simulink model "PasiveBalancer20S"  (R2021a)
settings: Solver=VariableStepAuto  StartTime=0.0  StopTime=30000  RelTol=1e-3
undefined symbols (not defined in the file): Ion, Lithium
libraries: spsIdealSwitchLib x22, spsSeriesRLCBranchLib x21, spsBatteryLib x20, spsDCVoltageSourceLib x1, spspowerguiLib x1
settings Model: SimulationMode=rapid-accelerator  Creator=jafar  LastModifiedBy=jafar
settings SolverCC: ZeroCrossAlgorithm=Adaptive
settings DebuggingCC: IgnoredZcDiagnostic=none

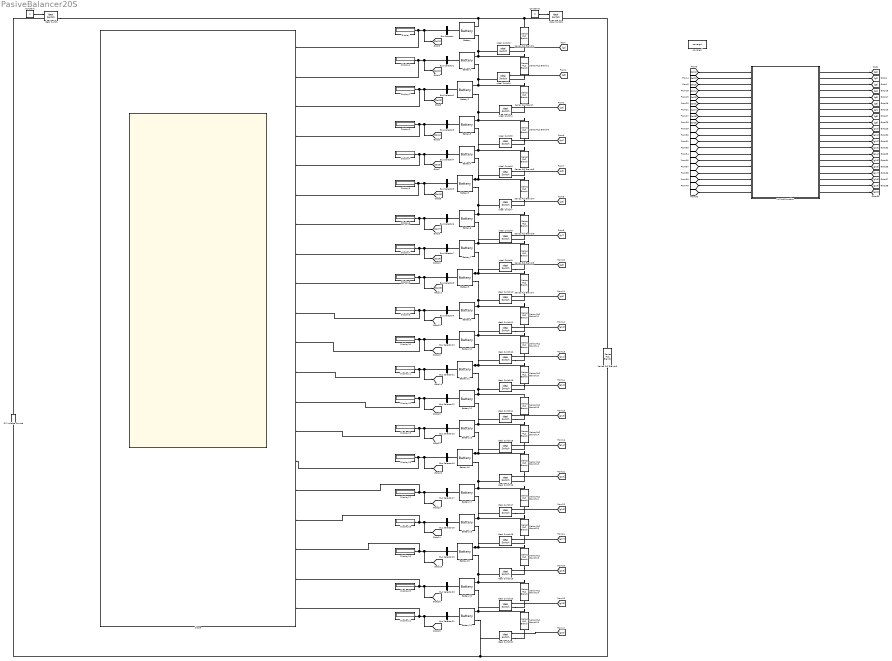
== system PasiveBalancer20S ==
  Battery : spsBatteryLib/Battery  BatType=Lithium-Ion  ShowTempParam=off  ThermalPreset=no  ShowAgeParam=off  NomV=3.7  NomQ=30  SOC=20  Batt_Tr=30  PresetModel=on  MaxQ=30  MinV=2.775  FullV=4.3068  Dis_rate=13.0435  R=0.0012333  Normal_OP=27.1304  expZone="[3.9974      1.4739]"  current=[6.5 13 32.5]  Units=Time  Tci=20  NomT=20  T2=-30  MaxQ2=4.8  FullV2=7.1  Normal_OP2=5.655  expZone2="[6.58           1]"  Rca=0.6  ti=2000  Dp=0  Neq0=0  Tsim=1e6  Ta1=25  Qeol=5.4*0.9  Reol=0.013333*1.2  Char_age=[2.3478, 3]  Dis_age=[2.3478, 10]  N1=1500  N2=10500  N3=1000  N4=1400  Ta2=45  N5=950
  Battery1 : spsBatteryLib/Battery  BatType=Lithium-Ion  ShowTempParam=off  ThermalPreset=no  ShowAgeParam=off  NomV=3.7  NomQ=30  SOC=23  Batt_Tr=30  PresetModel=on  MaxQ=30  MinV=2.775  FullV=4.3068  Dis_rate=13.0435  R=0.0012333  Normal_OP=27.1304  expZone="[3.9974      1.4739]"  current=[6.5 13 32.5]  Units=Time  Tci=20  NomT=20  T2=-30  MaxQ2=4.8  FullV2=7.1  Normal_OP2=5.655  expZone2="[6.58           1]"  Rca=0.6  ti=2000  Dp=0  Neq0=0  Tsim=1e6  Ta1=25  Qeol=5.4*0.9  Reol=0.013333*1.2  Char_age=[2.3478, 3]  Dis_age=[2.3478, 10]  N1=1500  N2=10500  N3=1000  N4=1400  Ta2=45  N5=950
  Battery10 : spsBatteryLib/Battery  BatType=Lithium-Ion  ShowTempParam=off  ThermalPreset=no  ShowAgeParam=off  NomV=3.7  NomQ=30  SOC=50  Batt_Tr=30  PresetModel=on  MaxQ=30  MinV=2.775  FullV=4.3068  Dis_rate=13.0435  R=0.0012333  Normal_OP=27.1304  expZone="[3.9974      1.4739]"  current=[6.5 13 32.5]  Units=Time  Tci=20  NomT=20  T2=-30  MaxQ2=4.8  FullV2=7.1  Normal_OP2=5.655  expZone2="[6.58           1]"  Rca=0.6  ti=2000  Dp=0  Neq0=0  Tsim=1e6  Ta1=25  Qeol=5.4*0.9  Reol=0.013333*1.2  Char_age=[2.3478, 3]  Dis_age=[2.3478, 10]  N1=1500  N2=10500  N3=1000  N4=1400  Ta2=45  N5=950
  Battery11 : spsBatteryLib/Battery  BatType=Lithium-Ion  ShowTempParam=off  ThermalPreset=no  ShowAgeParam=off  NomV=3.7  NomQ=30  SOC=53  Batt_Tr=30  PresetModel=on  MaxQ=30  MinV=2.775  FullV=4.3068  Dis_rate=13.0435  R=0.0012333  Normal_OP=27.1304  expZone="[3.9974      1.4739]"  current=[6.5 13 32.5]  Units=Time  Tci=20  NomT=20  T2=-30  MaxQ2=4.8  FullV2=7.1  Normal_OP2=5.655  expZone2="[6.58           1]"  Rca=0.6  ti=2000  Dp=0  Neq0=0  Tsim=1e6  Ta1=25  Qeol=5.4*0.9  Reol=0.013333*1.2  Char_age=[2.3478, 3]  Dis_age=[2.3478, 10]  N1=1500  N2=10500  N3=1000  N4=1400  Ta2=45  N5=950
  Battery12 : spsBatteryLib/Battery  BatType=Lithium-Ion  ShowTempParam=off  ThermalPreset=no  ShowAgeParam=off  NomV=3.7  NomQ=30  SOC=56  Batt_Tr=30  PresetModel=on  MaxQ=30  MinV=2.775  FullV=4.3068  Dis_rate=13.0435  R=0.0012333  Normal_OP=27.1304  expZone="[3.9974      1.4739]"  current=[6.5 13 32.5]  Units=Time  Tci=20  NomT=20  T2=-30  MaxQ2=4.8  FullV2=7.1  Normal_OP2=5.655  expZone2="[6.58           1]"  Rca=0.6  ti=2000  Dp=0  Neq0=0  Tsim=1e6  Ta1=25  Qeol=5.4*0.9  Reol=0.013333*1.2  Char_age=[2.3478, 3]  Dis_age=[2.3478, 10]  N1=1500  N2=10500  N3=1000  N4=1400  Ta2=45  N5=950
  Battery13 : spsBatteryLib/Battery  BatType=Lithium-Ion  ShowTempParam=off  ThermalPreset=no  ShowAgeParam=off  NomV=3.7  NomQ=30  SOC=59  Batt_Tr=30  PresetModel=on  MaxQ=30  MinV=2.775  FullV=4.3068  Dis_rate=13.0435  R=0.0012333  Normal_OP=27.1304  expZone="[3.9974      1.4739]"  current=[6.5 13 32.5]  Units=Time  Tci=20  NomT=20  T2=-30  MaxQ2=4.8  FullV2=7.1  Normal_OP2=5.655  expZone2="[6.58           1]"  Rca=0.6  ti=2000  Dp=0  Neq0=0  Tsim=1e6  Ta1=25  Qeol=5.4*0.9  Reol=0.013333*1.2  Char_age=[2.3478, 3]  Dis_age=[2.3478, 10]  N1=1500  N2=10500  N3=1000  N4=1400  Ta2=45  N5=950
  Battery16 : spsBatteryLib/Battery  BatType=Lithium-Ion  ShowTempParam=off  ThermalPreset=no  ShowAgeParam=off  NomV=3.7  NomQ=30  SOC=62  Batt_Tr=30  PresetModel=on  MaxQ=30  MinV=2.775  FullV=4.3068  Dis_rate=13.0435  R=0.0012333  Normal_OP=27.1304  expZone="[3.9974      1.4739]"  current=[6.5 13 32.5]  Units=Time  Tci=20  NomT=20  T2=-30  MaxQ2=4.8  FullV2=7.1  Normal_OP2=5.655  expZone2="[6.58           1]"  Rca=0.6  ti=2000  Dp=0  Neq0=0  Tsim=1e6  Ta1=25  Qeol=5.4*0.9  Reol=0.013333*1.2  Char_age=[2.3478, 3]  Dis_age=[2.3478, 10]  N1=1500  N2=10500  N3=1000  N4=1400  Ta2=45  N5=950
  Battery17 : spsBatteryLib/Battery  BatType=Lithium-Ion  ShowTempParam=off  ThermalPreset=no  ShowAgeParam=off  NomV=3.7  NomQ=30  SOC=65  Batt_Tr=30  PresetModel=on  MaxQ=30  MinV=2.775  FullV=4.3068  Dis_rate=13.0435  R=0.0012333  Normal_OP=27.1304  expZone="[3.9974      1.4739]"  current=[6.5 13 32.5]  Units=Time  Tci=20  NomT=20  T2=-30  MaxQ2=4.8  FullV2=7.1  Normal_OP2=5.655  expZone2="[6.58           1]"  Rca=0.6  ti=2000  Dp=0  Neq0=0  Tsim=1e6  Ta1=25  Qeol=5.4*0.9  Reol=0.013333*1.2  Char_age=[2.3478, 3]  Dis_age=[2.3478, 10]  N1=1500  N2=10500  N3=1000  N4=1400  Ta2=45  N5=950
  Battery18 : spsBatteryLib/Battery  BatType=Lithium-Ion  ShowTempParam=off  ThermalPreset=no  ShowAgeParam=off  NomV=3.7  NomQ=30  SOC=68  Batt_Tr=30  PresetModel=on  MaxQ=30  MinV=2.775  FullV=4.3068  Dis_rate=13.0435  R=0.0012333  Normal_OP=27.1304  expZone="[3.9974      1.4739]"  current=[6.5 13 32.5]  Units=Time  Tci=20  NomT=20  T2=-30  MaxQ2=4.8  FullV2=7.1  Normal_OP2=5.655  expZone2="[6.58           1]"  Rca=0.6  ti=2000  Dp=0  Neq0=0  Tsim=1e6  Ta1=25  Qeol=5.4*0.9  Reol=0.013333*1.2  Char_age=[2.3478, 3]  Dis_age=[2.3478, 10]  N1=1500  N2=10500  N3=1000  N4=1400  Ta2=45  N5=950
  Battery19 : spsBatteryLib/Battery  BatType=Lithium-Ion  ShowTempParam=off  ThermalPreset=no  ShowAgeParam=off  NomV=3.7  NomQ=30  SOC=71  Batt_Tr=30  PresetModel=on  MaxQ=30  MinV=2.775  FullV=4.3068  Dis_rate=13.0435  R=0.0012333  Normal_OP=27.1304  expZone="[3.9974      1.4739]"  current=[6.5 13 32.5]  Units=Time  Tci=20  NomT=20  T2=-30  MaxQ2=4.8  FullV2=7.1  Normal_OP2=5.655  expZone2="[6.58           1]"  Rca=0.6  ti=2000  Dp=0  Neq0=0  Tsim=1e6  Ta1=25  Qeol=5.4*0.9  Reol=0.013333*1.2  Char_age=[2.3478, 3]  Dis_age=[2.3478, 10]  N1=1500  N2=10500  N3=1000  N4=1400  Ta2=45  N5=950
  Battery2 : spsBatteryLib/Battery  BatType=Lithium-Ion  ShowTempParam=off  ThermalPreset=no  ShowAgeParam=off  NomV=3.7  NomQ=30  SOC=26  Batt_Tr=30  PresetModel=on  MaxQ=30  MinV=2.775  FullV=4.3068  Dis_rate=13.0435  R=0.0012333  Normal_OP=27.1304  expZone="[3.9974      1.4739]"  current=[6.5 13 32.5]  Units=Time  Tci=20  NomT=20  T2=-30  MaxQ2=4.8  FullV2=7.1  Normal_OP2=5.655  expZone2="[6.58           1]"  Rca=0.6  ti=2000  Dp=0  Neq0=0  Tsim=1e6  Ta1=25  Qeol=5.4*0.9  Reol=0.013333*1.2  Char_age=[2.3478, 3]  Dis_age=[2.3478, 10]  N1=1500  N2=10500  N3=1000  N4=1400  Ta2=45  N5=950
  Battery20 : spsBatteryLib/Battery  BatType=Lithium-Ion  ShowTempParam=off  ThermalPreset=no  ShowAgeParam=off  NomV=3.7  NomQ=30  SOC=74  Batt_Tr=30  PresetModel=on  MaxQ=30  MinV=2.775  FullV=4.3068  Dis_rate=13.0435  R=0.0012333  Normal_OP=27.1304  expZone="[3.9974      1.4739]"  current=[6.5 13 32.5]  Units=Time  Tci=20  NomT=20  T2=-30  MaxQ2=4.8  FullV2=7.1  Normal_OP2=5.655  expZone2="[6.58           1]"  Rca=0.6  ti=2000  Dp=0  Neq0=0  Tsim=1e6  Ta1=25  Qeol=5.4*0.9  Reol=0.013333*1.2  Char_age=[2.3478, 3]  Dis_age=[2.3478, 10]  N1=1500  N2=10500  N3=1000  N4=1400  Ta2=45  N5=950
  Battery21 : spsBatteryLib/Battery  BatType=Lithium-Ion  ShowTempParam=off  ThermalPreset=no  ShowAgeParam=off  NomV=3.7  NomQ=30  SOC=77  Batt_Tr=30  PresetModel=on  MaxQ=30  MinV=2.775  FullV=4.3068  Dis_rate=13.0435  R=0.0012333  Normal_OP=27.1304  expZone="[3.9974      1.4739]"  current=[6.5 13 32.5]  Units=Time  Tci=20  NomT=20  T2=-30  MaxQ2=4.8  FullV2=7.1  Normal_OP2=5.655  expZone2="[6.58           1]"  Rca=0.6  ti=2000  Dp=0  Neq0=0  Tsim=1e6  Ta1=25  Qeol=5.4*0.9  Reol=0.013333*1.2  Char_age=[2.3478, 3]  Dis_age=[2.3478, 10]  N1=1500  N2=10500  N3=1000  N4=1400  Ta2=45  N5=950
  Battery3 : spsBatteryLib/Battery  BatType=Lithium-Ion  ShowTempParam=off  ThermalPreset=no  ShowAgeParam=off  NomV=3.7  NomQ=30  SOC=29  Batt_Tr=30  PresetModel=on  MaxQ=30  MinV=2.775  FullV=4.3068  Dis_rate=13.0435  R=0.0012333  Normal_OP=27.1304  expZone="[3.9974      1.4739]"  current=[6.5 13 32.5]  Units=Time  Tci=20  NomT=20  T2=-30  MaxQ2=4.8  FullV2=7.1  Normal_OP2=5.655  expZone2="[6.58           1]"  Rca=0.6  ti=2000  Dp=0  Neq0=0  Tsim=1e6  Ta1=25  Qeol=5.4*0.9  Reol=0.013333*1.2  Char_age=[2.3478, 3]  Dis_age=[2.3478, 10]  N1=1500  N2=10500  N3=1000  N4=1400  Ta2=45  N5=950
  Battery4 : spsBatteryLib/Battery  BatType=Lithium-Ion  ShowTempParam=off  ThermalPreset=no  ShowAgeParam=off  NomV=3.7  NomQ=30  SOC=32  Batt_Tr=30  PresetModel=on  MaxQ=30  MinV=2.775  FullV=4.3068  Dis_rate=13.0435  R=0.0012333  Normal_OP=27.1304  expZone="[3.9974      1.4739]"  current=[6.5 13 32.5]  Units=Time  Tci=20  NomT=20  T2=-30  MaxQ2=4.8  FullV2=7.1  Normal_OP2=5.655  expZone2="[6.58           1]"  Rca=0.6  ti=2000  Dp=0  Neq0=0  Tsim=1e6  Ta1=25  Qeol=5.4*0.9  Reol=0.013333*1.2  Char_age=[2.3478, 3]  Dis_age=[2.3478, 10]  N1=1500  N2=10500  N3=1000  N4=1400  Ta2=45  N5=950
  Battery5 : spsBatteryLib/Battery  BatType=Lithium-Ion  ShowTempParam=off  ThermalPreset=no  ShowAgeParam=off  NomV=3.7  NomQ=30  SOC=35  Batt_Tr=30  PresetModel=on  MaxQ=30  MinV=2.775  FullV=4.3068  Dis_rate=13.0435  R=0.0012333  Normal_OP=27.1304  expZone="[3.9974      1.4739]"  current=[6.5 13 32.5]  Units=Time  Tci=20  NomT=20  T2=-30  MaxQ2=4.8  FullV2=7.1  Normal_OP2=5.655  expZone2="[6.58           1]"  Rca=0.6  ti=2000  Dp=0  Neq0=0  Tsim=1e6  Ta1=25  Qeol=5.4*0.9  Reol=0.013333*1.2  Char_age=[2.3478, 3]  Dis_age=[2.3478, 10]  N1=1500  N2=10500  N3=1000  N4=1400  Ta2=45  N5=950
  Battery6 : spsBatteryLib/Battery  BatType=Lithium-Ion  ShowTempParam=off  ThermalPreset=no  ShowAgeParam=off  NomV=3.7  NomQ=30  SOC=38  Batt_Tr=30  PresetModel=on  MaxQ=30  MinV=2.775  FullV=4.3068  Dis_rate=13.0435  R=0.0012333  Normal_OP=27.1304  expZone="[3.9974      1.4739]"  current=[6.5 13 32.5]  Units=Time  Tci=20  NomT=20  T2=-30  MaxQ2=4.8  FullV2=7.1  Normal_OP2=5.655  expZone2="[6.58           1]"  Rca=0.6  ti=2000  Dp=0  Neq0=0  Tsim=1e6  Ta1=25  Qeol=5.4*0.9  Reol=0.013333*1.2  Char_age=[2.3478, 3]  Dis_age=[2.3478, 10]  N1=1500  N2=10500  N3=1000  N4=1400  Ta2=45  N5=950
  Battery7 : spsBatteryLib/Battery  BatType=Lithium-Ion  ShowTempParam=off  ThermalPreset=no  ShowAgeParam=off  NomV=3.7  NomQ=30  SOC=41  Batt_Tr=30  PresetModel=on  MaxQ=30  MinV=2.775  FullV=4.3068  Dis_rate=13.0435  R=0.0012333  Normal_OP=27.1304  expZone="[3.9974      1.4739]"  current=[6.5 13 32.5]  Units=Time  Tci=20  NomT=20  T2=-30  MaxQ2=4.8  FullV2=7.1  Normal_OP2=5.655  expZone2="[6.58           1]"  Rca=0.6  ti=2000  Dp=0  Neq0=0  Tsim=1e6  Ta1=25  Qeol=5.4*0.9  Reol=0.013333*1.2  Char_age=[2.3478, 3]  Dis_age=[2.3478, 10]  N1=1500  N2=10500  N3=1000  N4=1400  Ta2=45  N5=950
  Battery8 : spsBatteryLib/Battery  BatType=Lithium-Ion  ShowTempParam=off  ThermalPreset=no  ShowAgeParam=off  NomV=3.7  NomQ=30  SOC=44  Batt_Tr=30  PresetModel=on  MaxQ=30  MinV=2.775  FullV=4.3068  Dis_rate=13.0435  R=0.0012333  Normal_OP=27.1304  expZone="[3.9974      1.4739]"  current=[6.5 13 32.5]  Units=Time  Tci=20  NomT=20  T2=-30  MaxQ2=4.8  FullV2=7.1  Normal_OP2=5.655  expZone2="[6.58           1]"  Rca=0.6  ti=2000  Dp=0  Neq0=0  Tsim=1e6  Ta1=25  Qeol=5.4*0.9  Reol=0.013333*1.2  Char_age=[2.3478, 3]  Dis_age=[2.3478, 10]  N1=1500  N2=10500  N3=1000  N4=1400  Ta2=45  N5=950
  Battery9 : spsBatteryLib/Battery  BatType=Lithium-Ion  ShowTempParam=off  ThermalPreset=no  ShowAgeParam=off  NomV=3.7  NomQ=30  SOC=47  Batt_Tr=30  PresetModel=on  MaxQ=30  MinV=2.775  FullV=4.3068  Dis_rate=13.0435  R=0.0012333  Normal_OP=27.1304  expZone="[3.9974      1.4739]"  current=[6.5 13 32.5]  Units=Time  Tci=20  NomT=20  T2=-30  MaxQ2=4.8  FullV2=7.1  Normal_OP2=5.655  expZone2="[6.58           1]"  Rca=0.6  ti=2000  Dp=0  Neq0=0  Tsim=1e6  Ta1=25  Qeol=5.4*0.9  Reol=0.013333*1.2  Char_age=[2.3478, 3]  Dis_age=[2.3478, 10]  N1=1500  N2=10500  N3=1000  N4=1400  Ta2=45  N5=950
  Bus Selector{,1..13,16..21} (20 alike) : BusSelector  OutputSignals=SOC (%)
  Constant : Constant
  Constant1 : Constant  Value=0
  DC Voltage Source : spsDCVoltageSourceLib/DC Voltage Source  Amplitude=84  Measurements=None
  Display{,1..13,16..21} (20 alike) : Display
  Ideal Switch{,1..21} (22 alike) : spsIdealSwitchLib/Ideal Switch  Ron=0.001  Lon=0  IC=0  Rs=1e5  Cs=inf  Measurements=on
  MATLAB Function : MATLAB Function  TreatAsAtomicUnit=on
  Scope : Scope  NumInputPorts=20
  Series RLC Branch{,1..2,4..14,18..21,23..24} (20 alike) : spsSeriesRLCBranchLib/Series RLC Branch  LConnTagsString=__new0  RConnTagsString=__new0  BranchType=R  Resistance=1  Inductance=1e-3  SetiL0=off  InitialCurrent=0  Capacitance=1e-6  Setx0=off  InitialVoltage=0  Measurements=None
  Series RLC Branch3 : spsSeriesRLCBranchLib/Series RLC Branch  LConnTagsString=__new0  RConnTagsString=__new0  BranchType=R  Resistance=1.73  Inductance=1e-3  SetiL0=off  InitialCurrent=0  Capacitance=1e-6  Setx0=off  InitialVoltage=0  Measurements=None
  powergui : spspowerguiLib/powergui  Priority=1  SimulationMode=Continuous  SampleTime=50e-6  frequency=60  Iterations=50  frequencyindice=0  Pbase=100e6  ErrMax=1e-4  UnitsV=kV  UnitsW=MW  buscounter=0  FunctionMessages=off  echomessages=off  EnableUseOfTLC=off  CurrentSourceSwitches=off  DisableSnubberDevices=off  DisableRonSwitches=off  DisableVfSwitches=off  DisplayEquations=off  AutomaticDiscreteSolvers=off  SolverType=Tustin/Backward Euler (TBE)  Interpol=off  ExternalGateDelay=off  methode=off  Ts=100  x0status=blocks  SPID=on  SwTol=0  HookPort=off  NonlinearTolerance=1e-4  nMaxIteration=100  ContinueOnMaxIteration=off  RestoreLinks=warning  ResistiveCurrentMeasurement=off  Frange=[0:2:500]  Ylog=off  Xlog=on  ShowGrid=off  save=off  variable=ZData  structure=0  ZoomFFT=off  StartTime=0.0  cycles=1  DisplayStyle=1  fundamental=60  FreqAxis=off  MaxFrequency=1000  frequencyindicesteady=1  RmsSteady=1  display=off
  wires:
  Constant/1 -> Ideal Switch/1
  Constant1/1 -> Ideal Switch1/1
  Battery/1 -> Bus Selector/1
  Battery1/1 -> Bus Selector1/1
  Battery2/1 -> Bus Selector2/1
  Bus Selector/1 -> [SoC1], Scope/1, Display/1  "<SOC (%)>"
  Bus Selector1/1 -> [SoC2], Scope/2, Display1/1  "<SOC (%)>"
  Bus Selector2/1 -> [SoC3], Scope/3, Display2/1  "<SOC (%)>"
  [g1] -> Ideal Switch2/1
  [g2] -> Ideal Switch3/1
  [SoC1] -> MATLAB Function/1(u1)
  [SoC2] -> MATLAB Function/2(u2)
  [SoC3] -> MATLAB Function/3(u3)
  Bus Selector5/1 -> [SoC6], Scope/6, Display5/1  "<SOC (%)>"
  Bus Selector3/1 -> [SoC4], Scope/4, Display3/1  "<SOC (%)>"
  Battery4/1 -> Bus Selector4/1
  Battery5/1 -> Bus Selector5/1
  Bus Selector4/1 -> [SoC5], Scope/5, Display4/1  "<SOC (%)>"
  Battery3/1 -> Bus Selector3/1
  Bus Selector8/1 -> [SoC9], Scope/9, Display8/1  "<SOC (%)>"
  Bus Selector6/1 -> [SoC7], Scope/7, Display6/1  "<SOC (%)>"
  Battery7/1 -> Bus Selector7/1
  Battery8/1 -> Bus Selector8/1
  Bus Selector7/1 -> [SoC8], Scope/8, Display7/1  "<SOC (%)>"
  Battery6/1 -> Bus Selector6/1
  Bus Selector11/1 -> [SoC12], Scope/12, Display11/1  "<SOC (%)>"
  [g10] -> Ideal Switch11/1
  Bus Selector9/1 -> [SoC10], Scope/10, Display9/1  "<SOC (%)>"
  Battery10/1 -> Bus Selector10/1
  Battery11/1 -> Bus Selector11/1
  Bus Selector10/1 -> [SoC11], Scope/11, Display10/1  "<SOC (%)>"
  [g12] -> Ideal Switch13/1
  Battery9/1 -> Bus Selector9/1
  Battery17/1 -> Bus Selector17/1
  [g18] -> Ideal Switch19/1
  Bus Selector17/1 -> [SoC16], Scope/16, Display17/1  "<SOC (%)>"
  Battery19/1 -> Bus Selector19/1
  Bus Selector18/1 -> [SoC17], Scope/17, Display18/1  "<SOC (%)>"
  Battery18/1 -> Bus Selector18/1
  [g16] -> Ideal Switch17/1
  Bus Selector21/1 -> [SoC20], Scope/20, Display21/1  "<SOC (%)>"
  Battery20/1 -> Bus Selector20/1
  [g19] -> Ideal Switch20/1
  Bus Selector20/1 -> [SoC19], Scope/19, Display20/1  "<SOC (%)>"
  Battery21/1 -> Bus Selector21/1
  [g20] -> Ideal Switch21/1
  Bus Selector16/1 -> [SoC15], Scope/15, Display16/1  "<SOC (%)>"
  [g14] -> Ideal Switch15/1
  [g17] -> Ideal Switch18/1
  Bus Selector19/1 -> [SoC18], Scope/18, Display19/1  "<SOC (%)>"
  Battery13/1 -> Bus Selector13/1
  Battery16/1 -> Bus Selector16/1
  Bus Selector12/1 -> [SoC13], Scope/13, Display12/1  "<SOC (%)>"
  Bus Selector13/1 -> [SoC14], Scope/14, Display13/1  "<SOC (%)>"
  [g15] -> Ideal Switch16/1
  Battery12/1 -> Bus Selector12/1
  [SoC6] -> MATLAB Function/6(u6)
  [SoC5] -> MATLAB Function/5(u5)
  [SoC4] -> MATLAB Function/4(u4)
  [SoC9] -> MATLAB Function/9(u9)
  [SoC8] -> MATLAB Function/8(u8)
  [SoC7] -> MATLAB Function/7(u7)
  [SoC12] -> MATLAB Function/12(u12)
  [SoC11] -> MATLAB Function/11(u11)
  [SoC10] -> MATLAB Function/10(u10)
  [SoC14] -> MATLAB Function/14(u14)
  [SoC13] -> MATLAB Function/13(u13)
  [SoC16] -> MATLAB Function/16(u16)
  [SoC15] -> MATLAB Function/15(u15)
  [SoC19] -> MATLAB Function/19(u19)
  [SoC18] -> MATLAB Function/18(u18)
  [SoC17] -> MATLAB Function/17(u17)
  [SoC20] -> MATLAB Function/20(u20)
  MATLAB Function/1(g1) -> [g1]
  MATLAB Function/2(g2) -> [g2]
  MATLAB Function/3(g3) -> [g3]
  MATLAB Function/4(g4) -> [g4]
  MATLAB Function/5(g5) -> [g5]
  MATLAB Function/6(g6) -> [g6]
  MATLAB Function/7(g7) -> [g7]
  MATLAB Function/8(g8) -> [g8]
  MATLAB Function/9(g9) -> [g9]
  MATLAB Function/10(g10) -> [g10]
  MATLAB Function/11(g11) -> [g11]
  MATLAB Function/12(g12) -> [g12]
  MATLAB Function/13(g13) -> [g13]
  MATLAB Function/14(g14) -> [g14]
  MATLAB Function/15(g15) -> [g15]
  MATLAB Function/16(g16) -> [g16]
  MATLAB Function/17(g17) -> [g17]
  MATLAB Function/18(g18) -> [g18]
  MATLAB Function/19(g19) -> [g19]
  MATLAB Function/20(g20) -> [g20]
  [g3] -> Ideal Switch4/1
  [g4] -> Ideal Switch5/1
  [g5] -> Ideal Switch6/1
  [g6] -> Ideal Switch7/1
  [g7] -> Ideal Switch8/1
  [g8] -> Ideal Switch9/1
  [g9] -> Ideal Switch10/1
  [g11] -> Ideal Switch12/1
  [g13] -> Ideal Switch14/1
  connections:
  Battery/LConn2 -- Ideal Switch2/RConn1 -- Series RLC Branch1/LConn1 -- Battery1/LConn1
  Battery1/LConn2 -- Series RLC Branch/LConn1 -- Battery2/LConn1 -- Ideal Switch3/RConn1
  Series RLC Branch1/RConn1 -- Ideal Switch3/LConn1
  Series RLC Branch2/RConn1 -- Ideal Switch2/LConn1
  Battery/LConn1 -- Ideal Switch/RConn1 -- Ideal Switch1/LConn1 -- Series RLC Branch2/LConn1
  Ideal Switch/LConn1 -- DC Voltage Source/RConn1
  Series RLC Branch3/LConn1 -- Ideal Switch1/RConn1
  Battery4/LConn1 -- Battery3/LConn2 -- Ideal Switch5/RConn1 -- Series RLC Branch5/LConn1
  Battery5/LConn1 -- Series RLC Branch4/LConn1 -- Battery4/LConn2 -- Ideal Switch6/RConn1
  Battery7/LConn1 -- Battery6/LConn2 -- Ideal Switch8/RConn1 -- Series RLC Branch8/LConn1
  Battery8/LConn1 -- Battery7/LConn2 -- Ideal Switch9/RConn1 -- Series RLC Branch7/LConn1
  Battery10/LConn1 -- Battery9/LConn2 -- Ideal Switch11/RConn1 -- Series RLC Branch11/LConn1
  Battery11/LConn1 -- Series RLC Branch10/LConn1 -- Battery10/LConn2 -- Ideal Switch12/RConn1
  Battery21/LConn1 -- Series RLC Branch23/LConn1 -- Battery20/LConn2 -- Ideal Switch20/RConn1
  Battery18/LConn1 -- Series RLC Branch20/LConn1 -- Battery17/LConn2 -- Ideal Switch17/RConn1
  Battery19/LConn1 -- Series RLC Branch19/LConn1 -- Battery18/LConn2 -- Ideal Switch18/RConn1
  Battery13/LConn1 -- Battery12/LConn2 -- Ideal Switch14/RConn1 -- Series RLC Branch14/LConn1
  Battery16/LConn1 -- Battery13/LConn2 -- Ideal Switch15/RConn1 -- Series RLC Branch13/LConn1
  Battery2/LConn2 -- Series RLC Branch6/LConn1 -- Battery3/LConn1 -- Ideal Switch4/RConn1
  Battery5/LConn2 -- Ideal Switch7/RConn1 -- Series RLC Branch9/LConn1 -- Battery6/LConn1
  Battery8/LConn2 -- Ideal Switch10/RConn1 -- Series RLC Branch12/LConn1 -- Battery9/LConn1
  Battery11/LConn2 -- Ideal Switch13/RConn1 -- Series RLC Branch18/LConn1 -- Battery12/LConn1
  Battery16/LConn2 -- Series RLC Branch21/LConn1 -- Battery17/LConn1 -- Ideal Switch16/RConn1
  Battery19/LConn2 -- Series RLC Branch24/LConn1 -- Battery20/LConn1 -- Ideal Switch19/RConn1
  Series RLC Branch3/RConn1 -- Battery21/LConn2 -- Ideal Switch21/RConn1 -- DC Voltage Source/LConn1
  Series RLC Branch/RConn1 -- Ideal Switch4/LConn1
  Series RLC Branch6/RConn1 -- Ideal Switch5/LConn1
  Series RLC Branch5/RConn1 -- Ideal Switch6/LConn1
  Series RLC Branch4/RConn1 -- Ideal Switch7/LConn1
  Series RLC Branch9/RConn1 -- Ideal Switch8/LConn1
  Ideal Switch9/LConn1 -- Series RLC Branch8/RConn1
  Series RLC Branch7/RConn1 -- Ideal Switch10/LConn1
  Ideal Switch11/LConn1 -- Series RLC Branch12/RConn1
  Ideal Switch12/LConn1 -- Series RLC Branch11/RConn1
  Series RLC Branch10/RConn1 -- Ideal Switch13/LConn1
  Ideal Switch14/LConn1 -- Series RLC Branch18/RConn1
  Series RLC Branch14/RConn1 -- Ideal Switch15/LConn1
  Series RLC Branch13/RConn1 -- Ideal Switch16/LConn1
  Ideal Switch17/LConn1 -- Series RLC Branch21/RConn1
  Series RLC Branch20/RConn1 -- Ideal Switch18/LConn1
  Series RLC Branch19/RConn1 -- Ideal Switch19/LConn1
  Ideal Switch20/LConn1 -- Series RLC Branch24/RConn1
  Ideal Switch21/LConn1 -- Series RLC Branch23/RConn1

== matlab function PasiveBalancer20S/MATLAB Function ==
  data: u1 input; g1 output; u2 input; u3 input; u4 input; u5 input; u6 input; u7 input; u8 input; u9 input; u10 input; u11 input; u12 input; u13 input; u14 input; u15 input; u16 input; u17 input; u18 input; u19 input; u20 input; g2 output; g3 output; g4 output; g5 output; g6 output; g7 output; g8 output; g9 output; g10 output; g11 output; g12 output; g13 output; g14 output; g15 output; g16 output; g17 output; g18 output; g19 output; g20 output
function [g1, g2, g3, g4, g5, g6, g7, g8, g9, g10, g11, g12, g13, g14, g15, g16, g17, g18, g19, g20] = fcn(u1, u2, u3, u4, u5, u6, u7, u8, u9, u10, u11, u12, u13, u14, u15, u16, u17, u18, u19, u20)
     % 1. Kalikan input dengan 1000
    datas = [u1, u2, u3, u4, u5, u6, u7, u8, u9, u10, u11, u12, u13, u14, u15, u16, u17, u18, u19, u20];
    % 2. Definisikan sebagai integer
    datas = int32(datas);
    output = zeros(size(datas));
    rata_rata = mean(datas);

    for i = 1:length(datas)
        if datas(i) > rata_rata
            output(i) = 1;
        else
            output(i) = 0;
        end
    end

    % Menghasilkan output sesuai dengan urutan input
    g1 = output(1);
    g2 = output(2);
    g3 = output(3);
    g4 = output(4);
    g5 = output(5);
    g6 = output(6);
    g7 = output(7);
    g8 = output(8);
    g9 = output(9);
    g10 = output(10);
    g11 = output(11);
    g12 = output(12);
    g13 = output(13);
    g14 = output(14);
    g15 = output(15);
    g16 = output(16);
    g17 = output(17);
    g18 = output(18);
    g19 = output(19);
    g20 = output(20);
end
